simulink model "npc_controller"  (R2022a)
settings: Solver=FixedStepDiscrete  StartTime=0.0  StopTime=20  RelTol=1e-3  EnableMultiTasking=on
undefined symbols (not defined in the file): CAN_O_INT, CANA_BASE, Down, GPTRIP1SEL, GPTRIP2SEL, GPTRIP3SEL, Tsw, TZ1, TZ2, TZ3, Up
libraries: simulink x147, hdlsllib x90, c2802xlib x34, c2837xDlib x20, c280xlib x12, canmsglib x9, c2838xlib x8, idelinklib_common x3, c2806xlib x2, slpidlib x2, c28004xlib x2, c281xlib x2
(part 10 of 42)

== system npc_controller/CONTROL/STATE-MACHINE/CPU_CONTROL_750_precharge_pfc_ok2/updateSequencePhA ==
  note: Notes:
      | vac_adc = vac_actual*0.00264706+1.65
      | iac_adc = iac_actual*0.02+1.65
      | vbulk_adc = vbulk_actual*3.49e-3
      | vmid_adc = vmid_acutal*3.49e-3
  note: Note:
      | Vmid         C2
      | Vbulk        A5
      |
      | Va            A2/B6
      | Vb            B0
      | Vc            C0
      |
      | Ia             A3
      | Ib             A10/B1, C10
      | Ic             C1
  vxn : Inport
  ix : Inport  Port=2
  f : TriggerPort  TriggerType=function-call  VariantControl=(inherit)
      settings: CopyFcn=Stateflow.SLINSF.SimulinkMan.removeBlockPreDeleteFcn  PreDeleteFcn=Stateflow.SLINSF.SimulinkMan.unsafePredeleteFcn
  Cast To Single : DataTypeConversion  Commented=on  OutDataTypeStr=single  SaturateOnIntegerOverflow=off  RndMeth=Floor
  Cast To Single1 : DataTypeConversion  Commented=on  OutDataTypeStr=single  SaturateOnIntegerOverflow=off  RndMeth=Floor
  From5 : From  Commented=on  GotoTag=vxn
  From6 : From  Commented=on  GotoTag=pol_vxn
  From7 : From  Commented=on  GotoTag=ix
  From8 : From  Commented=on  GotoTag=pol_ix
  Function-Call Generator : simulink/Ports & Subsystems/Function-Call Generator  sample_time=-1  numberOfIterations=1  DisallowWideOutput=off
  Function-Call Split : FunctionCallSplit  NumOutputPorts=2
  Function-Call Split2 : FunctionCallSplit  NumOutputPorts=2
  Gain2 : Gain  Commented=on  Gain=200
  Gain3 : Gain  Commented=on  Gain=200
  Mux : Mux  Commented=on  Inputs=2
  Mux1 : Mux  Commented=on  Inputs=2
  Scope : Scope  Commented=on  NumInputPorts=3
  pol_final1 : Subsystem  Commented=on
  pol_ix1 : Subsystem  Commented=on
  pol_vxn1 : Subsystem
  vx_seq : Outport
  wires:
  pol_vxn1/1(pol_vxn) -> [pol_vxn]
  [pol_vxn] -> vx_seq/1
  Gain3/1 -> Mux1/2
  Cast To Single1/1 -> Gain3/1
  Gain2/1 -> Mux/2
  From7/1 -> Mux1/1
  From5/1 -> Mux/1
  ix/1 -> [ix]
  Cast To Single/1 -> Gain2/1
  From8/1 -> Cast To Single1/1
  From6/1 -> Cast To Single/1
  Mux1/1 -> Scope/2
  Mux/1 -> Scope/1
  pol_final1/1(pol) -> Scope/3
  [pol_ix] -> pol_final1/2(ix)
  [pol_vxn] -> pol_final1/1(vxn)
  pol_ix1/1(pol_ix) -> [pol_ix]
  [ix] -> pol_ix1/1(ix)
  [vxn] -> pol_vxn1/1(vxn)
  Function-Call Split2/2 -> Function-Call Split/1
  Function-Call Generator/1 -> Function-Call Split2/1
  Function-Call Split/1 -> pol_ix1/Trigger
  Function-Call Split2/1 -> pol_vxn1/Trigger
  Function-Call Split/2 -> pol_final1/Trigger
  vxn/1 -> [vxn]

== system npc_controller/CONTROL/STATE-MACHINE/CPU_CONTROL_750_precharge_pfc_ok2/updateSequencePhB ==
  note: Note:
      |
      | Function PWM # GPIO # LAUNCHPAD PIN #
      |
      | Synci EPWM1A GPIO0 J4.40
      | EPWM1B GPIO1 J4.39
      |
      | ORPS EPMW2A GPIO2 J4.38
      | EPWM2B GPIO3 J4.37
      |
      | RELAY EPWM3A GPIO4 J4.36
      |
      | TZ GPIO62 XX
      |
      | a_s1 EPWM6A GPIO10 J8.76
      | a_s2 EPWM7B GPIO13 XX
      | a_s3 EPWM6B GPIO11 J8.75
      | a_s4 EPWM7A GPIO12 XX
      |
      | b_s1 EPWM8B GPIO15 J8.73
      | b_s2 EPWM9B GPIO17 XX
      | b_s3 EPWM8A GPIO14 J8.74
      | b_s4 EPWM9A GPIO16 J4.33
      |
      | c_s1 EPWM10B GPIO19 J1.3
      | c_s2 EPWM11B GPIO21 XX
      | c_s3 EPWM10A GPIO18 J1.4
      | c_s4 EPWM11A GPIO20 XX
  note: Notes:
      | vac_adc = vac_actual*0.00264706+1.65
      | iac_adc = iac_actual*0.02+1.65
      | vbulk_adc = vbulk_actual*3.49e-3
      | vmid_adc = vmid_acutal*3.49e-3
  note: Note:
      | Vmid         C2
      | Vbulk        A5
      |
      | Va            A2/B6
      | Vb            B0
      | Vc            C0
      |
      | Ia             A3
      | Ib             A10/B1, C10
      | Ic             C1
  vxn : Inport
  ix : Inport  Port=2
  f : TriggerPort  TriggerType=function-call  VariantControl=(inherit)
      settings: CopyFcn=Stateflow.SLINSF.SimulinkMan.removeBlockPreDeleteFcn  PreDeleteFcn=Stateflow.SLINSF.SimulinkMan.unsafePredeleteFcn
  Cast To Single : DataTypeConversion  Commented=on  OutDataTypeStr=single  SaturateOnIntegerOverflow=off  RndMeth=Floor
  Cast To Single1 : DataTypeConversion  Commented=on  OutDataTypeStr=single  SaturateOnIntegerOverflow=off  RndMeth=Floor
  From5 : From  Commented=on  GotoTag=vxn
  From6 : From  Commented=on  GotoTag=pol_vxn
  From7 : From  Commented=on  GotoTag=ix
  From8 : From  Commented=on  GotoTag=pol_ix
  Function-Call Generator : simulink/Ports & Subsystems/Function-Call Generator  sample_time=-1  numberOfIterations=1  DisallowWideOutput=off
  Function-Call Split : FunctionCallSplit  NumOutputPorts=2
  Function-Call Split2 : FunctionCallSplit  NumOutputPorts=2
  Gain2 : Gain  Commented=on  Gain=200
  Gain3 : Gain  Commented=on  Gain=200
  Mux : Mux  Commented=on  Inputs=2
  Mux1 : Mux  Commented=on  Inputs=2
  Scope : Scope  Commented=on  NumInputPorts=3
  pol_final1 : Subsystem  Commented=on
  pol_ix1 : Subsystem  Commented=on
  pol_vxn1 : Subsystem
  vx_seq : Outport
  wires:
  pol_vxn1/1(pol_vxn) -> [pol_vxn]
  [pol_vxn] -> vx_seq/1
  Gain3/1 -> Mux1/2
  Cast To Single1/1 -> Gain3/1
  Gain2/1 -> Mux/2
  From7/1 -> Mux1/1
  From5/1 -> Mux/1
  ix/1 -> [ix]
  Cast To Single/1 -> Gain2/1
  From8/1 -> Cast To Single1/1
  From6/1 -> Cast To Single/1
  Mux1/1 -> Scope/2
  Mux/1 -> Scope/1
  pol_final1/1(pol) -> Scope/3
  [pol_ix] -> pol_final1/2(ix)
  [pol_vxn] -> pol_final1/1(vxn)
  pol_ix1/1(pol_ix) -> [pol_ix]
  [ix] -> pol_ix1/1(ix)
  [vxn] -> pol_vxn1/1(vxn)
  Function-Call Split2/2 -> Function-Call Split/1
  Function-Call Generator/1 -> Function-Call Split2/1
  Function-Call Split/1 -> pol_ix1/Trigger
  Function-Call Split2/1 -> pol_vxn1/Trigger
  Function-Call Split/2 -> pol_final1/Trigger
  vxn/1 -> [vxn]

== system npc_controller/CONTROL/STATE-MACHINE/CPU_CONTROL_750_precharge_pfc_ok2/updateSequencePhC ==
  note: Note:
      |
      | Function PWM # GPIO # LAUNCHPAD PIN #
      |
      | Synci EPWM1A GPIO0 J4.40
      | EPWM1B GPIO1 J4.39
      |
      | ORPS EPMW2A GPIO2 J4.38
      | EPWM2B GPIO3 J4.37
      |
      | RELAY EPWM3A GPIO4 J4.36
      |
      | TZ GPIO62 XX
      |
      | a_s1 EPWM6A GPIO10 J8.76
      | a_s2 EPWM7B GPIO13 XX
      | a_s3 EPWM6B GPIO11 J8.75
      | a_s4 EPWM7A GPIO12 XX
      |
      | b_s1 EPWM8B GPIO15 J8.73
      | b_s2 EPWM9B GPIO17 XX
      | b_s3 EPWM8A GPIO14 J8.74
      | b_s4 EPWM9A GPIO16 J4.33
      |
      | c_s1 EPWM10B GPIO19 J1.3
      | c_s2 EPWM11B GPIO21 XX
      | c_s3 EPWM10A GPIO18 J1.4
      | c_s4 EPWM11A GPIO20 XX
  note: Notes:
      | vac_adc = vac_actual*0.00264706+1.65
      | iac_adc = iac_actual*0.02+1.65
      | vbulk_adc = vbulk_actual*3.49e-3
      | vmid_adc = vmid_acutal*3.49e-3
  note: Note:
      | Vmid         C2
      | Vbulk        A5
      |
      | Va            A2/B6
      | Vb            B0
      | Vc            C0
      |
      | Ia             A3
      | Ib             A10/B1, C10
      | Ic             C1
  vxn : Inport
  ix : Inport  Port=2
  f : TriggerPort  TriggerType=function-call  VariantControl=(inherit)
      settings: CopyFcn=Stateflow.SLINSF.SimulinkMan.removeBlockPreDeleteFcn  PreDeleteFcn=Stateflow.SLINSF.SimulinkMan.unsafePredeleteFcn
  Cast To Single : DataTypeConversion  Commented=on  OutDataTypeStr=single  SaturateOnIntegerOverflow=off  RndMeth=Floor
  Cast To Single1 : DataTypeConversion  Commented=on  OutDataTypeStr=single  SaturateOnIntegerOverflow=off  RndMeth=Floor
  From5 : From  Commented=on  GotoTag=vxn
  From6 : From  Commented=on  GotoTag=pol_vxn
  From7 : From  Commented=on  GotoTag=ix
  From8 : From  Commented=on  GotoTag=pol_ix
  Function-Call Generator : simulink/Ports & Subsystems/Function-Call Generator  sample_time=-1  numberOfIterations=1  DisallowWideOutput=off
  Function-Call Split : FunctionCallSplit  NumOutputPorts=2
  Function-Call Split2 : FunctionCallSplit  NumOutputPorts=2
  Gain2 : Gain  Commented=on  Gain=200
  Gain3 : Gain  Commented=on  Gain=200
  Mux : Mux  Commented=on  Inputs=2
  Mux1 : Mux  Commented=on  Inputs=2
  Scope : Scope  Commented=on  NumInputPorts=3
  pol_final1 : Subsystem  Commented=on
  pol_ix1 : Subsystem  Commented=on
  pol_vxn1 : Subsystem
  vx_seq : Outport
  wires:
  [pol_vxn] -> vx_seq/1
  Gain3/1 -> Mux1/2
  Cast To Single1/1 -> Gain3/1
  Gain2/1 -> Mux/2
  From7/1 -> Mux1/1
  From5/1 -> Mux/1
  ix/1 -> [ix]
  Cast To Single/1 -> Gain2/1
  From8/1 -> Cast To Single1/1
  From6/1 -> Cast To Single/1
  Mux1/1 -> Scope/2
  Mux/1 -> Scope/1
  pol_final1/1(pol) -> Scope/3
  [pol_ix] -> pol_final1/2(ix)
  [pol_vxn] -> pol_final1/1(vxn)
  pol_ix1/1(pol_ix) -> [pol_ix]
  [ix] -> pol_ix1/1(ix)
  pol_vxn1/1(pol_vxn) -> [pol_vxn]
  [vxn] -> pol_vxn1/1(vxn)
  Function-Call Split2/2 -> Function-Call Split/1
  Function-Call Generator/1 -> Function-Call Split2/1
  Function-Call Split/1 -> pol_ix1/Trigger
  Function-Call Split2/1 -> pol_vxn1/Trigger
  Function-Call Split/2 -> pol_final1/Trigger
  vxn/1 -> [vxn]

== system npc_controller/CONTROL/STATE-MACHINE/If Action Subsystem ==
  Action Port : ActionPort
  Constant3 : Constant  Value=0  OutDataTypeStr=single  SampleTime=-1
  Out1 : Outport
  wires:
  Constant3/1 -> Out1/1

== system npc_controller/CONTROL/STATE-MACHINE/If Action Subsystem1 ==
  Action Port : ActionPort
  Constant3 : Constant  Value=2048  OutDataTypeStr=single  SampleTime=-1
  Out1 : Outport
  wires:
  Constant3/1 -> Out1/1

== system npc_controller/CONTROL/STATE-MACHINE/PLL ==
  note: Voltage-Controlled Oscillator (VCO)
  note: Loop Filter (LF)
  note: Phase Detector (PD)
  vxn : Inport  OutDataTypeStr=single
  Data Store Write : DataStoreWrite  Commented=on  DataStoreName=theta  IndexOptions=Index vector (dialog)  Indices=1  OutputSizes=1
  Delay1 : Delay  DelayLength=1  StateName=mem2
  Delay2 : Delay  DelayLength=1  StateName=mem1
  Gain : Gain  Commented=on  Gain=100  ParamDataTypeStr=uint16  OutDataTypeStr=uint16
  Gain4 : Gain  Gain=1/(2*pi)  ParamDataTypeStr=single  OutDataTypeStr=single
  Integrator2 : Subsystem
  Product : Product  OutDataTypeStr=single
  Product1 : Product  OutDataTypeStr=single
  Product2 : Product  OutDataTypeStr=single
  Scope1 : Scope  NumInputPorts=3
  Scope2 : Scope  NumInputPorts=4
  Scope4 : Scope  NumInputPorts=3
  Scope5 : Scope  NumInputPorts=3
  Subsystem1 : Subsystem
  Subsystem2 : Subsystem
  Sum : Sum  Inputs=|+-  AccumDataTypeStr=single  OutDataTypeStr=single
  Trigonometric Function1 : Trigonometry  Operator=sincos
  freq1 : Outport  VectorParamsAs1DForOutWhenUnconnected=off
  angle : Outport  Port=2  VectorParamsAs1DForOutWhenUnconnected=off
  mag1 : Outport  Port=3  VectorParamsAs1DForOutWhenUnconnected=off
  wires:
  Integrator2/1(theta) -> Scope2/3, angle/1, Gain/1, Delay1/1
  Subsystem1/1(y) -> mag1/1, Scope2/4, Product1/1, Scope4/1
  Sum/1 -> Scope1/3, Product2/1, Scope5/1, Delay2/1
  Gain4/1 -> freq1/1, Scope2/2
  Gain/1 -> Data Store Write/1
  vxn/1 -> Scope2/1, Scope1/1, Sum/1
  Product/1 -> Subsystem1/1(u)
  Product1/1 -> Scope4/3, Scope1/2, Sum/2
  Trigonometric Function1/2 -> Scope5/2, Product2/2
  Delay2/1 -> Product/1
  Subsystem2/1(y) -> Gain4/1, Integrator2/1(omega)
  Product2/1 -> Subsystem2/1(u), Scope5/3
  Delay1/1 -> Trigonometric Function1/1
  Trigonometric Function1/1 -> Scope4/2, Product1/2, Product/2

== system npc_controller/CONTROL/STATE-MACHINE/Subsystem1 ==
  adc : Inport
  Less Than : RelationalOperator  Operator=>  OutDataTypeStr=boolean  RndMeth=Simplest  InputSameDT=off
  Less Than1 : RelationalOperator  Operator=<  OutDataTypeStr=boolean  RndMeth=Simplest  InputSameDT=off
  Offset7 : Constant  Value=0  OutDataTypeStr=single
  Offset8 : Constant  Value=0  OutDataTypeStr=single
  Product : Product  OutDataTypeStr=single
  Product1 : Product  OutDataTypeStr=single
  vabc7 : Sum  Inputs=|+-  AccumDataTypeStr=single  OutDataTypeStr=single
  adc_rect : Outport
  wires:
  vabc7/1 -> adc_rect/1
  adc/1 -> Less Than/1, Product/1, Less Than1/1, Product1/1
  Product1/1 -> vabc7/2
  Product/1 -> vabc7/1
  Less Than/1 -> Product/2
  Offset8/1 -> Less Than1/2
  Offset7/1 -> Less Than/2
  Less Than1/1 -> Product1/2

== system npc_controller/CONTROL/STATE-MACHINE/Update_PFC_EN ==
  Dig_Input : Inport  OutDataTypeStr=boolean
  Constant : Constant  Value=67  OutDataTypeStr=uint16
  Constant1 : Constant  Value=67  OutDataTypeStr=uint16
  Constant2 : Constant  OutDataTypeStr=boolean
  Validate_DI : MATLABSystem  System=Validate_DI  SimulateUsing=Code generation
      mask Type: Validate_DI
      mask Display:
      | disp('Validate_DI');
      | port_label('input',1,'din');
      | port_label('input',2,'assert_logic');
      | port_label('input',3,'assert_dly');
      | port_label('input',4,'deassert_dly');
      | port_label('output',1,'status');
  Dig_Input_State : Outport  OutDataTypeStr=boolean
  wires:
  Constant1/1 -> Validate_DI/4
  Constant/1 -> Validate_DI/3
  Dig_Input/1 -> Validate_DI/1
  Constant2/1 -> Validate_DI/2
  Validate_DI/1 -> Dig_Input_State/1

== system npc_controller/CONTROL/SVPWM/IIR Filter1 ==
  x[n] : Inport
  1 - Lambda : Gain  Gain=1 - 0.98
  Delay : Delay  DelayLength=1
  Lambda : Gain  Gain=0.98
  Sum : Sum  Inputs=|++
  y[n] : Outport
  wires:
  x[n]/1 -> 1 - Lambda/1
  1 - Lambda/1 -> Sum/1
  Sum/1 -> Delay/1, y[n]/1
  Lambda/1 -> Sum/2
  Delay/1 -> Lambda/1

== system npc_controller/CONTROL/SVPWM/IIR Filter2 ==
  x[n] : Inport
  1 - Lambda : Gain  Gain=1 - 0.98
  Delay : Delay  DelayLength=1
  Lambda : Gain  Gain=0.98
  Sum : Sum  Inputs=|++
  y[n] : Outport
  wires:
  Delay/1 -> Lambda/1
  Lambda/1 -> Sum/2
  Sum/1 -> y[n]/1, Delay/1
  1 - Lambda/1 -> Sum/1
  x[n]/1 -> 1 - Lambda/1

== system npc_controller/CONTROL/SVPWM/PLL_Block ==
  abc : Inport
  Demux : Demux  Commented=on  Outputs=3
  If1 : If  Commented=on  IfExpression=(u1 > 0)  ShowElse=off
  SRF_PLL : Subsystem
  Subsystem : Subsystem  Commented=on
  theta : Outport  OutDataTypeStr=single
  wires:
  Demux/1 -> Subsystem/1(In1)
  abc/1 -> Demux/1, SRF_PLL/1(Vabc)
  Subsystem/1(Out1) -> If1/1
  SRF_PLL/3(theta) -> theta/1

== system npc_controller/CONTROL/SVPWM/SVPWM Generator (3-Level)1 ==
  Vabc_ref : Inport
  Vdc_P0 : Inport  Port=2
  Vdc_0N : Inport  Port=3
  Idc : Inport  Port=4
  Kp : Inport  Port=5
  Fsw : Inport  Port=6
  Neutral Point Voltage Deviation Control System : Subsystem
  Selector2 : Selector  InputPortWidth=2  IndexOptions=Index vector (dialog)  Indices=1  OutputSizes=1
  Timing Calculation : Subsystem
  TgABC_On : Outport
  TgABC_Off : Outport  Port=2
  Sn : Outport  Port=3
  wires:
  Fsw/1 -> Timing Calculation/3(Fsw)
  Kp/1 -> Neutral Point Voltage Deviation Control System/4(Kp)
  Vdc_0N/1 -> Neutral Point Voltage Deviation Control System/2(Vdc_0N)
  Vabc_ref/1 -> Timing Calculation/1(Uref)
  Neutral Point Voltage Deviation Control System/1(Out) -> Timing Calculation/2(DeltaVdc)
  Timing Calculation/3(Sn) -> Selector2/1
  Selector2/1 -> Sn/1
  Timing Calculation/1(TgABC_On) -> TgABC_On/1
  Timing Calculation/2(TgABC_Off) -> TgABC_Off/1
  Idc/1 -> Neutral Point Voltage Deviation Control System/3(Idc)
  Vdc_P0/1 -> Neutral Point Voltage Deviation Control System/1(Vdc_P0)

== system npc_controller/CONTROL/SVPWM/SVPWM2/calcCmpBal ==
  r_seq : Inport  OutDataTypeStr=double  PortDimensions=4
  s_seq : Inport  Port=2  OutDataTypeStr=double  PortDimensions=4
  t_seq : Inport  Port=3  OutDataTypeStr=double  PortDimensions=4
  Tx : Inport  Port=4  OutDataTypeStr=double  PortDimensions=1
  Ty : Inport  Port=5  OutDataTypeStr=double  PortDimensions=1
  Tz : Inport  Port=6  OutDataTypeStr=double  PortDimensions=1
  vbal_coef : Inport  Port=7
  f : TriggerPort  TriggerType=function-call  VariantControl=(inherit)
      settings: CopyFcn=Stateflow.SLINSF.SimulinkMan.removeBlockPreDeleteFcn  PreDeleteFcn=Stateflow.SLINSF.SimulinkMan.unsafePredeleteFcn
  Add : Sum  Inputs=++++
  Add1 : Sum  Inputs=++++
  Add2 : Sum  Inputs=++++
  Constant : Constant
  Demux : Demux
  Demux1 : Demux
  Demux2 : Demux
  Display : Display
  Display1 : Display
  Gain1 : Gain  Gain=1/15e-6
  Gain11 : Gain  Gain=1/15e-6
  Gain6 : Gain  Gain=1/15e-6
  Product{,1..17} (18 alike) : Product
  Subtract : Sum  Inputs=+-
  cmp_r : Outport
  cmp_s : Outport  Port=2
  cmp_t : Outport  Port=3
  wires:
  [vbal_coef_n] -> Product14/2
  [vbal_coef_p] -> Product15/2
  [vbal_coef_p] -> Product17/2
  [vbal_coef_n] -> Product16/2
  [vbal_coef_n] -> Product13/2
  [vbal_coef_p] -> Product12/2
  vbal_coef/1 -> [vbal_coef_p], Display1/1, Subtract/2
  Subtract/1 -> [vbal_coef_n], Display/1
  Constant/1 -> Subtract/1
  Tz/1 -> [Tz]
  s_seq/1 -> [s_seq]
  t_seq/1 -> [t_seq]
  Gain11/1 -> cmp_t/1
  Product17/1 -> Product11/2
  [Ty] -> Product10/2
  [Tx] -> Product9/2
  Demux2/4 -> Product11/1
  Demux2/3 -> Product10/1
  Demux2/2 -> Product9/1
  Product11/1 -> Add2/4
  Product10/1 -> Add2/3
  Product9/1 -> Add2/2
  Demux2/1 -> Product8/1
  Product16/1 -> Product8/2
  Product8/1 -> Add2/1
  [Tz] -> Product17/1
  Add2/1 -> Gain11/1
  [Tz] -> Product16/1
  [t_seq] -> Demux2/1
  Gain6/1 -> cmp_s/1
  [s_seq] -> Demux1/1
  [Tz] -> Product14/1
  Add1/1 -> Gain6/1
  [Tz] -> Product15/1
  Product4/1 -> Add1/1
  Product14/1 -> Product4/2
  Demux1/1 -> Product4/1
  Product5/1 -> Add1/2
  Product6/1 -> Add1/3
  Product7/1 -> Add1/4
  Demux1/2 -> Product5/1
  Demux1/3 -> Product6/1
  Demux1/4 -> Product7/1
  [Tx] -> Product5/2
  [Ty] -> Product6/2
  Product15/1 -> Product7/2
  Product12/1 -> Product3/2
  [Ty] -> Product2/2
  [Tx] -> Product1/2
  Demux/4 -> Product3/1
  Demux/3 -> Product2/1
  Demux/2 -> Product1/1
  Product3/1 -> Add/4
  Product2/1 -> Add/3
  Product1/1 -> Add/2
  Demux/1 -> Product/1
  Product13/1 -> Product/2
  Product/1 -> Add/1
  [Tz] -> Product12/1
  Gain1/1 -> cmp_r/1
  Add/1 -> Gain1/1
  [Tz] -> Product13/1
  [r_seq] -> Demux/1
  Tx/1 -> [Tx]
  Ty/1 -> [Ty]
  r_seq/1 -> [r_seq]

== system npc_controller/CONTROL/SVPWM/SVPWM2/calcDwellingTimes ==
  Tsw : Inport  OutDataTypeStr=double  PortDimensions=1
  vref_fict_mag_alpha : Inport  Port=2  OutDataTypeStr=double  PortDimensions=1
  vref_fict_mag_beta : Inport  Port=3  OutDataTypeStr=double  PortDimensions=1
  vx_fict_mag_alpha : Inport  Port=4  OutDataTypeStr=double  PortDimensions=1
  vx_fict_mag_beta : Inport  Port=5  OutDataTypeStr=double  PortDimensions=1
  vy_fict_mag_alpha : Inport  Port=6  OutDataTypeStr=double  PortDimensions=1
  vy_fict_mag_beta : Inport  Port=7  OutDataTypeStr=double  PortDimensions=1
  f : TriggerPort  TriggerType=function-call  VariantControl=(inherit)
      settings: CopyFcn=Stateflow.SLINSF.SimulinkMan.removeBlockPreDeleteFcn  PreDeleteFcn=Stateflow.SLINSF.SimulinkMan.unsafePredeleteFcn
  Add : Sum  Inputs=+-
  Add1 : Sum  Inputs=+--
  Cast To Single : DataTypeConversion  OutDataTypeStr=single  SaturateOnIntegerOverflow=off  RndMeth=Floor
  Cast To Single1 : DataTypeConversion  OutDataTypeStr=single  SaturateOnIntegerOverflow=off  RndMeth=Floor
  Cast To Single2 : DataTypeConversion  OutDataTypeStr=single  SaturateOnIntegerOverflow=off  RndMeth=Floor
  Display{,1..17} (18 alike) : Display
  Divide : Product  Inputs=**/
  Divide1 : Product  Inputs=*/
  Product{,1..5} (6 alike) : Product
  Subtract : Sum  Inputs=+-
  Subtract1 : Sum  Inputs=+-
  Tx : Outport
  Ty : Outport  Port=2
  Tz : Outport  Port=3
  wires:
  Add1/1 -> Display3/1, Cast To Single2/1
  Divide1/1 -> Display2/1, [Ty], Cast To Single1/1
  Divide/1 -> Cast To Single/1, Display1/1, [Tx]
  Tsw/1 -> Display4/1, [Tsw]
  vref_fict_mag_alpha/1 -> Display5/1, [vref_fict_mag_alpha]
  vref_fict_mag_beta/1 -> Display6/1, [vref_fict_mag_beta]
  vx_fict_mag_alpha/1 -> Display7/1, [vx_fict_mag_alpha]
  vx_fict_mag_beta/1 -> Display8/1, [vx_fict_mag_beta]
  vy_fict_mag_alpha/1 -> Display9/1, [vy_fict_mag_alpha]
  vy_fict_mag_beta/1 -> Display10/1, [vy_fict_mag_beta]
  [vref_fict_mag_beta] -> Product/1
  [vy_fict_mag_alpha] -> Product/2
  [vref_fict_mag_alpha] -> Product1/1
  [vy_fict_mag_beta] -> Product1/2
  [vx_fict_mag_alpha] -> Product3/1
  [vy_fict_mag_beta] -> Product3/2
  Product/1 -> Add/1, Display12/1
  Product1/1 -> Add/2, Display13/1
  Product2/1 -> Subtract/1, Display15/1
  Product3/1 -> Subtract/2, Display14/1
  Add/1 -> Divide/2, Display11/1
  Subtract/1 -> Divide/3, Display16/1
  Product4/1 -> Display/1, Subtract1/1
  [vref_fict_mag_alpha] -> Product4/1
  [Tsw] -> Product4/2
  [vx_fict_mag_alpha] -> Product5/1
  [Tx] -> Product5/2
  Product5/1 -> Subtract1/2
  Subtract1/1 -> Divide1/1
  [vy_fict_mag_alpha] -> Divide1/2
  [Ty] -> Add1/3
  [Tx] -> Add1/2
  [Tsw] -> Add1/1
  Cast To Single/1 -> Tx/1
  Cast To Single1/1 -> Ty/1
  Cast To Single2/1 -> Tz/1
  [Tsw] -> Divide/1, Display17/1
  [vy_fict_mag_alpha] -> Product2/2
  [vx_fict_mag_beta] -> Product2/1

== system npc_controller/CONTROL/SVPWM/SVPWM2/detSeq ==
  subsector : Inport  OutDataTypeStr=double  PortDimensions=1
  f : TriggerPort  TriggerType=function-call  VariantControl=(inherit)
      settings: CopyFcn=Stateflow.SLINSF.SimulinkMan.removeBlockPreDeleteFcn  PreDeleteFcn=Stateflow.SLINSF.SimulinkMan.unsafePredeleteFcn
  Cast To Double : DataTypeConversion  OutDataTypeStr=double  SaturateOnIntegerOverflow=off  RndMeth=Floor
  Cast To Double1 : DataTypeConversion  OutDataTypeStr=double  SaturateOnIntegerOverflow=off  RndMeth=Floor
  Cast To Double2 : DataTypeConversion  OutDataTypeStr=double  SaturateOnIntegerOverflow=off  RndMeth=Floor
  Constant{,5,7..8,12,17} (6 alike) : Constant  Value=[0 1 1 1]
  Constant1 : Constant  Value=[0 1 0 1]
  Constant{2..3,10..11,14..15} (6 alike) : Constant  Value=[0 0 0 1]
  Constant13 : Constant  Value=[0 1 0 1]
  Constant16 : Constant  Value=[0 0 1 1]
  Constant18 : Constant  Commented=on  Value=[1 1 0 0]
  Constant19 : Constant  Commented=on  Value=[1 0 0 0]
  Constant20 : Constant  Commented=on  Value=[1 1 1 0]
  Constant21 : Constant  Commented=on  Value=[1 1 1 0]
  Constant22 : Constant  Commented=on  Value=[1 1 0 0]
  Constant23 : Constant  Commented=on  Value=[1 0 0 0]
  Constant24 : Constant  Commented=on  Value=[1 0 0 0]
  Constant25 : Constant  Commented=on  Value=[1 1 1 0]
  Constant26 : Constant  Commented=on  Value=[1 1 0 0]
  Constant4 : Constant  Value=[0 0 1 1]
  Constant6 : Constant  Value=[0 0 1 1]
  Constant9 : Constant  Value=[0 1 0 1]
  Multiport Switch : MultiPortSwitch  Inputs=6  DataPortForDefault=Additional data port  SaturateOnIntegerOverflow=off  InputSameDT=off
  Multiport Switch1 : MultiPortSwitch  Inputs=6  DataPortForDefault=Additional data port  SaturateOnIntegerOverflow=off  InputSameDT=off
  Multiport Switch2 : MultiPortSwitch  Inputs=6  DataPortForDefault=Additional data port  SaturateOnIntegerOverflow=off  InputSameDT=off
  r_seq : Outport
  s_seq : Outport  Port=2
  t_seq : Outport  Port=3
  wires:
  Multiport Switch2/1 -> Cast To Double2/1
  Constant15/1 -> Multiport Switch2/3
  Constant16/1 -> Multiport Switch2/4
  Constant17/1 -> Multiport Switch2/5
  Constant12/1 -> Multiport Switch2/6
  Constant13/1 -> Multiport Switch2/7
  Constant14/1 -> Multiport Switch2/2
  [subsector] -> Multiport Switch2/1
  Multiport Switch1/1 -> Cast To Double1/1
  [subsector] -> Multiport Switch1/1
  Constant6/1 -> Multiport Switch1/2
  Constant11/1 -> Multiport Switch1/7
  Constant10/1 -> Multiport Switch1/6
  Constant9/1 -> Multiport Switch1/5
  Constant8/1 -> Multiport Switch1/4
  Constant7/1 -> Multiport Switch1/3
  Constant1/1 -> Multiport Switch/3
  Constant2/1 -> Multiport Switch/4
  Constant3/1 -> Multiport Switch/5
  Constant4/1 -> Multiport Switch/6
  Constant5/1 -> Multiport Switch/7
  Constant/1 -> Multiport Switch/2
  [subsector] -> Multiport Switch/1
  subsector/1 -> [subsector]
  Multiport Switch/1 -> Cast To Double/1
  Cast To Double/1 -> r_seq/1
  Cast To Double1/1 -> s_seq/1
  Cast To Double2/1 -> t_seq/1

== system npc_controller/CONTROL/SVPWM/SVPWM_with_bal/calcCmp ==
  r_seq : Inport  OutDataTypeStr=double  PortDimensions=4
  s_seq : Inport  Port=2  OutDataTypeStr=double  PortDimensions=4
  t_seq : Inport  Port=3  OutDataTypeStr=double  PortDimensions=4
  Tx : Inport  Port=4  OutDataTypeStr=double  PortDimensions=1
  Ty : Inport  Port=5  OutDataTypeStr=double  PortDimensions=1
  Tz : Inport  Port=6  OutDataTypeStr=double  PortDimensions=1
  f : TriggerPort  TriggerType=function-call  VariantControl=(inherit)
      settings: CopyFcn=Stateflow.SLINSF.SimulinkMan.removeBlockPreDeleteFcn  PreDeleteFcn=Stateflow.SLINSF.SimulinkMan.unsafePredeleteFcn
  Add : Sum  Inputs=++++
  Add1 : Sum  Inputs=++++
  Add2 : Sum  Inputs=++++
  Demux : Demux
  Demux1 : Demux
  Demux2 : Demux
  Gain{,2,5,7,10,12} (6 alike) : Gain  Gain=0.5
  Gain1 : Gain  Gain=1/15e-6
  Gain11 : Gain  Gain=1/15e-6
  Gain6 : Gain  Gain=1/15e-6
  Product{,1..11} (12 alike) : Product
  cmp_r : Outport
  cmp_s : Outport  Port=2
  cmp_t : Outport  Port=3
  wires:
  r_seq/1 -> [r_seq]
  Ty/1 -> [Ty]
  Tx/1 -> [Tx]
  Tz/1 -> [Tz]
  [r_seq] -> Demux/1
  [Tz] -> Gain/1
  Add/1 -> Gain1/1
  Gain1/1 -> cmp_r/1
  [Tz] -> Gain2/1
  Product/1 -> Add/1
  Gain/1 -> Product/2
  Demux/1 -> Product/1
  Product1/1 -> Add/2
  Product2/1 -> Add/3
  Product3/1 -> Add/4
  Demux/2 -> Product1/1
  Demux/3 -> Product2/1
  Demux/4 -> Product3/1
  [Tx] -> Product1/2
  [Ty] -> Product2/2
  Gain2/1 -> Product3/2
  Gain7/1 -> Product7/2
  [Ty] -> Product6/2
  [Tx] -> Product5/2
  Demux1/4 -> Product7/1
  Demux1/3 -> Product6/1
  Demux1/2 -> Product5/1
  Product7/1 -> Add1/4
  Product6/1 -> Add1/3
  Product5/1 -> Add1/2
  Demux1/1 -> Product4/1
  Gain5/1 -> Product4/2
  Product4/1 -> Add1/1
  [Tz] -> Gain7/1
  Add1/1 -> Gain6/1
  [Tz] -> Gain5/1
  [s_seq] -> Demux1/1
  Gain6/1 -> cmp_s/1
  [t_seq] -> Demux2/1
  [Tz] -> Gain10/1
  Add2/1 -> Gain11/1
  [Tz] -> Gain12/1
  Product8/1 -> Add2/1
  Gain10/1 -> Product8/2
  Demux2/1 -> Product8/1
  Product9/1 -> Add2/2
  Product10/1 -> Add2/3
  Product11/1 -> Add2/4
  Demux2/2 -> Product9/1
  Demux2/3 -> Product10/1
  Demux2/4 -> Product11/1
  [Tx] -> Product9/2
  [Ty] -> Product10/2
  Gain12/1 -> Product11/2
  Gain11/1 -> cmp_t/1
  t_seq/1 -> [t_seq]
  s_seq/1 -> [s_seq]

== system npc_controller/CONTROL/SVPWM/SVPWM_with_bal/calcCmpWithBal ==
  r_seq : Inport  OutDataTypeStr=double  PortDimensions=4
  s_seq : Inport  Port=2  OutDataTypeStr=double  PortDimensions=4
  t_seq : Inport  Port=3  OutDataTypeStr=double  PortDimensions=4
  Tx : Inport  Port=4  OutDataTypeStr=double  PortDimensions=1
  Ty : Inport  Port=5  OutDataTypeStr=double  PortDimensions=1
  Tz : Inport  Port=6  OutDataTypeStr=double  PortDimensions=1
  f : TriggerPort  TriggerType=function-call  VariantControl=(inherit)
      settings: CopyFcn=Stateflow.SLINSF.SimulinkMan.removeBlockPreDeleteFcn  PreDeleteFcn=Stateflow.SLINSF.SimulinkMan.unsafePredeleteFcn
  Add : Sum  Inputs=++++
  Add1 : Sum  Inputs=++++
  Add2 : Sum  Inputs=++++
  Demux : Demux
  Demux1 : Demux
  Demux2 : Demux
  Gain{,2,5,7,10,12} (6 alike) : Gain  Gain=0.5
  Gain1 : Gain  Gain=1/15e-6
  Gain11 : Gain  Gain=1/15e-6
  Gain6 : Gain  Gain=1/15e-6
  Product{,1..11} (12 alike) : Product
  cmp_r : Outport
  cmp_s : Outport  Port=2
  cmp_t : Outport  Port=3
  wires:
  r_seq/1 -> [r_seq]
  Ty/1 -> [Ty]
  Tx/1 -> [Tx]
  Tz/1 -> [Tz]
  [r_seq] -> Demux/1
  [Tz] -> Gain/1
  Add/1 -> Gain1/1
  Gain1/1 -> cmp_r/1
  [Tz] -> Gain2/1
  Product/1 -> Add/1
  Gain/1 -> Product/2
  Demux/1 -> Product/1
  Product1/1 -> Add/2
  Product2/1 -> Add/3
  Product3/1 -> Add/4
  Demux/2 -> Product1/1
  Demux/3 -> Product2/1
  Demux/4 -> Product3/1
  [Tx] -> Product1/2
  [Ty] -> Product2/2
  Gain2/1 -> Product3/2
  Gain7/1 -> Product7/2
  [Ty] -> Product6/2
  [Tx] -> Product5/2
  Demux1/4 -> Product7/1
  Demux1/3 -> Product6/1
  Demux1/2 -> Product5/1
  Product7/1 -> Add1/4
  Product6/1 -> Add1/3
  Product5/1 -> Add1/2
  Demux1/1 -> Product4/1
  Gain5/1 -> Product4/2
  Product4/1 -> Add1/1
  [Tz] -> Gain7/1
  Add1/1 -> Gain6/1
  [Tz] -> Gain5/1
  [s_seq] -> Demux1/1
  Gain6/1 -> cmp_s/1
  [t_seq] -> Demux2/1
  [Tz] -> Gain10/1
  Add2/1 -> Gain11/1
  [Tz] -> Gain12/1
  Product8/1 -> Add2/1
  Gain10/1 -> Product8/2
  Demux2/1 -> Product8/1
  Product9/1 -> Add2/2
  Product10/1 -> Add2/3
  Product11/1 -> Add2/4
  Demux2/2 -> Product9/1
  Demux2/3 -> Product10/1
  Demux2/4 -> Product11/1
  [Tx] -> Product9/2
  [Ty] -> Product10/2
  Gain12/1 -> Product11/2
  Gain11/1 -> cmp_t/1
  t_seq/1 -> [t_seq]
  s_seq/1 -> [s_seq]

== system npc_controller/CONTROL/SVPWM/SVPWM_with_bal/calcDwellingTimes ==
  Tsw : Inport  OutDataTypeStr=double  PortDimensions=1
  vref_fict_mag_alpha : Inport  Port=2  OutDataTypeStr=double  PortDimensions=1
  vref_fict_mag_beta : Inport  Port=3  OutDataTypeStr=double  PortDimensions=1
  vx_fict_mag_alpha : Inport  Port=4  OutDataTypeStr=double  PortDimensions=1
  vx_fict_mag_beta : Inport  Port=5  OutDataTypeStr=double  PortDimensions=1
  vy_fict_mag_alpha : Inport  Port=6  OutDataTypeStr=double  PortDimensions=1
  vy_fict_mag_beta : Inport  Port=7  OutDataTypeStr=double  PortDimensions=1
  f : TriggerPort  TriggerType=function-call  VariantControl=(inherit)
      settings: CopyFcn=Stateflow.SLINSF.SimulinkMan.removeBlockPreDeleteFcn  PreDeleteFcn=Stateflow.SLINSF.SimulinkMan.unsafePredeleteFcn
  Add : Sum  Inputs=+-
  Add1 : Sum  Inputs=+--
  Cast To Single : DataTypeConversion  OutDataTypeStr=single  SaturateOnIntegerOverflow=off  RndMeth=Floor
  Cast To Single1 : DataTypeConversion  OutDataTypeStr=single  SaturateOnIntegerOverflow=off  RndMeth=Floor
  Cast To Single2 : DataTypeConversion  OutDataTypeStr=single  SaturateOnIntegerOverflow=off  RndMeth=Floor
  Display{,1..17} (18 alike) : Display
  Divide : Product  Inputs=**/
  Divide1 : Product  Inputs=*/
  Product{,1..5} (6 alike) : Product
  Subtract : Sum  Inputs=+-
  Subtract1 : Sum  Inputs=+-
  Tx : Outport
  Ty : Outport  Port=2
  Tz : Outport  Port=3
  wires:
  [vx_fict_mag_beta] -> Product2/1
  [vy_fict_mag_alpha] -> Product2/2
  [Tsw] -> Display17/1, Divide/1
  Cast To Single2/1 -> Tz/1
  Cast To Single1/1 -> Ty/1
  Cast To Single/1 -> Tx/1
  [Tsw] -> Add1/1
  [Tx] -> Add1/2
  [Ty] -> Add1/3
  [vy_fict_mag_alpha] -> Divide1/2
  Subtract1/1 -> Divide1/1
  Product5/1 -> Subtract1/2
  [Tx] -> Product5/2
  [vx_fict_mag_alpha] -> Product5/1
  [Tsw] -> Product4/2
  [vref_fict_mag_alpha] -> Product4/1
  Product4/1 -> Subtract1/1, Display/1
  Subtract/1 -> Display16/1, Divide/3
  Add/1 -> Display11/1, Divide/2
  Product3/1 -> Display14/1, Subtract/2
  Product2/1 -> Display15/1, Subtract/1
  Product1/1 -> Display13/1, Add/2
  Product/1 -> Display12/1, Add/1
  [vy_fict_mag_beta] -> Product3/2
  [vx_fict_mag_alpha] -> Product3/1
  [vy_fict_mag_beta] -> Product1/2
  [vref_fict_mag_alpha] -> Product1/1
  [vy_fict_mag_alpha] -> Product/2
  [vref_fict_mag_beta] -> Product/1
  vy_fict_mag_beta/1 -> [vy_fict_mag_beta], Display10/1
  vy_fict_mag_alpha/1 -> [vy_fict_mag_alpha], Display9/1
  vx_fict_mag_beta/1 -> [vx_fict_mag_beta], Display8/1
  vx_fict_mag_alpha/1 -> [vx_fict_mag_alpha], Display7/1
  vref_fict_mag_beta/1 -> [vref_fict_mag_beta], Display6/1
  vref_fict_mag_alpha/1 -> [vref_fict_mag_alpha], Display5/1
  Tsw/1 -> [Tsw], Display4/1
  Divide/1 -> [Tx], Display1/1, Cast To Single/1
  Divide1/1 -> Cast To Single1/1, [Ty], Display2/1
  Add1/1 -> Cast To Single2/1, Display3/1

== system npc_controller/CONTROL/SVPWM/SVPWM_with_bal/detSeq ==
  subsector : Inport  OutDataTypeStr=double  PortDimensions=1
  f : TriggerPort  TriggerType=function-call  VariantControl=(inherit)
      settings: CopyFcn=Stateflow.SLINSF.SimulinkMan.removeBlockPreDeleteFcn  PreDeleteFcn=Stateflow.SLINSF.SimulinkMan.unsafePredeleteFcn
  Cast To Double : DataTypeConversion  OutDataTypeStr=double  SaturateOnIntegerOverflow=off  RndMeth=Floor
  Cast To Double1 : DataTypeConversion  OutDataTypeStr=double  SaturateOnIntegerOverflow=off  RndMeth=Floor
  Cast To Double2 : DataTypeConversion  OutDataTypeStr=double  SaturateOnIntegerOverflow=off  RndMeth=Floor
  Constant : Constant  Value=[0 1 1 1]
  Constant1 : Constant  Value=[1 1 0 0]
  Constant10 : Constant  Value=[0 0 0 1]
  Constant11 : Constant  Value=[1 0 0 0]
  Constant12 : Constant  Value=[0 1 1 1]
  Constant13 : Constant  Value=[1 1 0 0]
  Constant14 : Constant  Value=[0 0 0 1]
  Constant15 : Constant  Value=[1 0 0 0]
  Constant16 : Constant  Value=[0 0 1 1]
  Constant17 : Constant  Value=[1 1 1 0]
  Constant2 : Constant  Value=[0 0 0 1]
  Constant3 : Constant  Value=[1 0 0 0]
  Constant4 : Constant  Value=[0 0 1 1]
  Constant5 : Constant  Value=[1 1 1 0]
  Constant6 : Constant  Value=[0 0 1 1]
  Constant7 : Constant  Value=[1 1 1 0]
  Constant8 : Constant  Value=[0 1 1 1]
  Constant9 : Constant  Value=[1 1 0 0]
  Multiport Switch : MultiPortSwitch  Inputs=6  DataPortForDefault=Additional data port  SaturateOnIntegerOverflow=off  InputSameDT=off
  Multiport Switch1 : MultiPortSwitch  Inputs=6  DataPortForDefault=Additional data port  SaturateOnIntegerOverflow=off  InputSameDT=off
  Multiport Switch2 : MultiPortSwitch  Inputs=6  DataPortForDefault=Additional data port  SaturateOnIntegerOverflow=off  InputSameDT=off
  r_seq : Outport
  s_seq : Outport  Port=2
  t_seq : Outport  Port=3
  wires:
  Cast To Double2/1 -> t_seq/1
  Cast To Double1/1 -> s_seq/1
  Cast To Double/1 -> r_seq/1
  Multiport Switch/1 -> Cast To Double/1
  subsector/1 -> [subsector]
  [subsector] -> Multiport Switch/1
  Constant/1 -> Multiport Switch/2
  Constant5/1 -> Multiport Switch/7
  Constant4/1 -> Multiport Switch/6
  Constant3/1 -> Multiport Switch/5
  Constant2/1 -> Multiport Switch/4
  Constant1/1 -> Multiport Switch/3
  Constant7/1 -> Multiport Switch1/3
  Constant8/1 -> Multiport Switch1/4
  Constant9/1 -> Multiport Switch1/5
  Constant10/1 -> Multiport Switch1/6
  Constant11/1 -> Multiport Switch1/7
  Constant6/1 -> Multiport Switch1/2
  [subsector] -> Multiport Switch1/1
  Multiport Switch1/1 -> Cast To Double1/1
  [subsector] -> Multiport Switch2/1
  Constant14/1 -> Multiport Switch2/2
  Constant13/1 -> Multiport Switch2/7
  Constant12/1 -> Multiport Switch2/6
  Constant17/1 -> Multiport Switch2/5
  Constant16/1 -> Multiport Switch2/4
  Constant15/1 -> Multiport Switch2/3
  Multiport Switch2/1 -> Cast To Double2/1

== system npc_controller/CONTROL/SVPWM/SVPWM_with_bal/detSeqFixedSmallVector ==
  subsector : Inport  OutDataTypeStr=double  PortDimensions=1
  f : TriggerPort  TriggerType=function-call  VariantControl=(inherit)
      settings: CopyFcn=Stateflow.SLINSF.SimulinkMan.removeBlockPreDeleteFcn  PreDeleteFcn=Stateflow.SLINSF.SimulinkMan.unsafePredeleteFcn
  Cast To Double : DataTypeConversion  OutDataTypeStr=double  SaturateOnIntegerOverflow=off  RndMeth=Floor
  Cast To Double1 : DataTypeConversion  OutDataTypeStr=double  SaturateOnIntegerOverflow=off  RndMeth=Floor
  Cast To Double2 : DataTypeConversion  OutDataTypeStr=double  SaturateOnIntegerOverflow=off  RndMeth=Floor
  Constant{,7..8,12,17} (5 alike) : Constant  Value=[0 1 1 1]
  Constant1 : Constant  Value=[1 1 0 0]
  Constant{2,10..11,14..15} (5 alike) : Constant  Value=[0 0 0 1]
  Constant13 : Constant  Value=[0 1 0 1]
  Constant16 : Constant  Value=[0 0 1 1]
  Constant18 : Constant  Commented=on  Value=[1 1 0 0]
  Constant19 : Constant  Commented=on  Value=[1 0 0 0]
  Constant20 : Constant  Commented=on  Value=[1 1 1 0]
  Constant21 : Constant  Commented=on  Value=[1 1 1 0]
  Constant22 : Constant  Commented=on  Value=[1 1 0 0]
  Constant23 : Constant  Commented=on  Value=[1 0 0 0]
  Constant24 : Constant  Commented=on  Value=[1 0 0 0]
  Constant25 : Constant  Commented=on  Value=[1 1 1 0]
  Constant26 : Constant  Commented=on  Value=[1 1 0 0]
  Constant3 : Constant  Value=[1 0 0 0]
  Constant4 : Constant  Value=[0 0 1 1]
  Constant5 : Constant  Value=[1 1 1 0]
  Constant6 : Constant  Value=[0 0 1 1]
  Constant9 : Constant  Value=[0 1 0 1]
  Multiport Switch : MultiPortSwitch  Inputs=6  DataPortForDefault=Additional data port  SaturateOnIntegerOverflow=off  InputSameDT=off
  Multiport Switch1 : MultiPortSwitch  Inputs=6  DataPortForDefault=Additional data port  SaturateOnIntegerOverflow=off  InputSameDT=off
  Multiport Switch2 : MultiPortSwitch  Inputs=6  DataPortForDefault=Additional data port  SaturateOnIntegerOverflow=off  InputSameDT=off
  r_seq : Outport
  s_seq : Outport  Port=2
  t_seq : Outport  Port=3
  wires:
  Cast To Double2/1 -> t_seq/1
  Cast To Double1/1 -> s_seq/1
  Cast To Double/1 -> r_seq/1
  Multiport Switch/1 -> Cast To Double/1
  subsector/1 -> [subsector]
  [subsector] -> Multiport Switch/1
  Constant/1 -> Multiport Switch/2
  Constant5/1 -> Multiport Switch/7
  Constant4/1 -> Multiport Switch/6
  Constant3/1 -> Multiport Switch/5
  Constant2/1 -> Multiport Switch/4
  Constant1/1 -> Multiport Switch/3
  Constant7/1 -> Multiport Switch1/3
  Constant8/1 -> Multiport Switch1/4
  Constant9/1 -> Multiport Switch1/5
  Constant10/1 -> Multiport Switch1/6
  Constant11/1 -> Multiport Switch1/7
  Constant6/1 -> Multiport Switch1/2
  [subsector] -> Multiport Switch1/1
  Multiport Switch1/1 -> Cast To Double1/1
  [subsector] -> Multiport Switch2/1
  Constant14/1 -> Multiport Switch2/2
  Constant13/1 -> Multiport Switch2/7
  Constant12/1 -> Multiport Switch2/6
  Constant17/1 -> Multiport Switch2/5
  Constant16/1 -> Multiport Switch2/4
  Constant15/1 -> Multiport Switch2/3
  Multiport Switch2/1 -> Cast To Double2/1

== system npc_controller/CONTROL/SVPWM/Subsystem ==
  Trigger : TriggerPort  TriggerType=function-call  VariantControl=Variant  PortDimensions=1
  Constant16 : Constant
  Out1 : Outport
  wires:
  Constant16/1 -> Out1/1

== system npc_controller/CONTROL/SVPWM/Subsystem1 ==
  note: interacting PID
  error : Inport
  disable : Inport  Port=2
  Constant : Constant  Value=18.57
  Constant1 : Constant  Value=-34.95
  Constant2 : Constant  Value=470
  Constant3 : Constant  Value=-470
  Constant4 : Constant  Value=16.46
  Constant5 : Constant  Value=-1.246
  Constant6 : Constant  Value=0.2457
  Delay{1..4} (4 alike) : Delay  DelayLength=1  InitialCondition=0  ExternalReset=Level
      settings: InputPortMap=u0,r5
  Product{1..5} (5 alike) : Product
  Saturation Dynamic1 : simulink/Discontinuities/Saturation Dynamic  OutMin=[]  OutMax=[]  OutDataTypeStr=double  OutputDataTypeScalingMode=double  OutDataType=fixdt(1, 16)  OutScaling=2^-10  DoSatur=off
  Scope : Scope  NumInputPorts=4
  Sum : Sum  Inputs=|+++--
  pi : Outport
  wires:
  [error] -> Scope/1  "error"
  [kP_term] -> Scope/2  "kP_term"
  [kI_term] -> Scope/3  "kI_term"
  [pi] -> Scope/4  "PI"
  [a0] -> Product3/2
  Sum/1 -> Saturation Dynamic1/2
  [integ_min] -> Saturation Dynamic1/3
  [integ_max] -> Saturation Dynamic1/1
  Constant2/1 -> [integ_max]
  Constant3/1 -> [integ_min]
  Constant1/1 -> [a1]
  error/1 -> [error]
  [a1] -> Product2/2
  Constant/1 -> [a0]
  [error] -> Delay2/1, Product3/1
  Delay2/1 -> Product2/1, Delay3/1
  Saturation Dynamic1/1 -> pi/1, Delay1/1, [pi]
  Delay3/1 -> Product1/1
  [a2] -> Product1/2
  Product3/1 -> Sum/1
  Product2/1 -> Sum/2
  Product1/1 -> Sum/3
  Delay1/1 -> Product4/2, Delay4/1
  [b1] -> Product4/1
  Delay4/1 -> Product5/2
  Product5/1 -> Sum/5
  Product4/1 -> Sum/4
  [b2] -> Product5/1
  Constant5/1 -> [b1]
  Constant4/1 -> [a2]
  Constant6/1 -> [b2]
  disable/1 -> Delay4/2, Delay1/2, Delay3/2, Delay2/2

== system npc_controller/CONTROL/SVPWM/Subsystem2 ==
  note: Parallel PI
  error : Inport
  Constant : Constant  Value=0.3055
  Constant1 : Constant  Value=-0.3052
  Constant2 : Constant  Value=50
  Constant3 : Constant  Value=-50
  Constant4 : Constant  Commented=on  Value=36
  Constant5 : Constant  Commented=on  Value=-36
  Constant6 : Constant  Commented=on  Value=0.611
  Constant7 : Constant  Commented=on  Value=-0.6105
  Delay1 : Delay  DelayLength=1  InitialCondition=22
  Delay2 : Delay  DelayLength=1  InitialCondition=0
  Product2 : Product
  Product3 : Product
  Saturation Dynamic1 : simulink/Discontinuities/Saturation Dynamic  OutMin=[]  OutMax=[]  OutDataTypeStr=double  OutputDataTypeScalingMode=double  OutDataType=fixdt(1, 16)  OutScaling=2^-10  DoSatur=off
  Scope : Scope  NumInputPorts=4
  Sum : Sum  Inputs=|++
  Sum3 : Sum  Inputs=|++
  pi : Outport
  wires:
  Saturation Dynamic1/1 -> [pi], Delay1/1, pi/1
  Delay2/1 -> Product2/1
  [error] -> Delay2/1
  Sum3/1 -> Sum/2, [kI_term]
  Delay1/1 -> Sum3/2
  Constant/1 -> [kp]
  [ki] -> Product2/2
  error/1 -> [error]
  Constant1/1 -> [ki]
  [error] -> Product3/1
  Product3/1 -> [kP_term], Sum/1
  Product2/1 -> Sum3/1
  Constant3/1 -> [integ_min]
  Constant2/1 -> [integ_max]
  [integ_max] -> Saturation Dynamic1/1
  [integ_min] -> Saturation Dynamic1/3
  Sum/1 -> Saturation Dynamic1/2
  [kp] -> Product3/2
  [pi] -> Scope/4  "PI"
  [kI_term] -> Scope/3  "kI_term"
  [kP_term] -> Scope/2  "kP_term"
  [error] -> Scope/1  "error"

== system npc_controller/CONTROL/SVPWM/Subsystem4 ==
  note: interacting PID
  error : Inport
  disable : Inport  Port=2
  Constant : Constant  Value=18.57
  Constant1 : Constant  Value=-34.95
  Constant2 : Constant  Value=470
  Constant3 : Constant  Value=-470
  Constant4 : Constant  Value=16.46
  Constant5 : Constant  Value=-1.246
  Constant6 : Constant  Value=0.2457
  Delay{1..4} (4 alike) : Delay  DelayLength=1  InitialCondition=0  ExternalReset=Level
      settings: InputPortMap=u0,r5
  Product{1..5} (5 alike) : Product
  Saturation Dynamic1 : simulink/Discontinuities/Saturation Dynamic  OutMin=[]  OutMax=[]  OutDataTypeStr=double  OutputDataTypeScalingMode=double  OutDataType=fixdt(1, 16)  OutScaling=2^-10  DoSatur=off
  Scope : Scope  NumInputPorts=4
  Sum : Sum  Inputs=|+++--
  pi : Outport
  wires:
  disable/1 -> Delay2/2, Delay3/2, Delay1/2, Delay4/2
  Constant6/1 -> [b2]
  Constant4/1 -> [a2]
  Constant5/1 -> [b1]
  [b2] -> Product5/1
  Product4/1 -> Sum/4
  Product5/1 -> Sum/5
  Delay4/1 -> Product5/2
  [b1] -> Product4/1
  Delay1/1 -> Delay4/1, Product4/2
  Product1/1 -> Sum/3
  Product2/1 -> Sum/2
  Product3/1 -> Sum/1
  [a2] -> Product1/2
  Delay3/1 -> Product1/1
  Saturation Dynamic1/1 -> [pi], Delay1/1, pi/1
  Delay2/1 -> Delay3/1, Product2/1
  [error] -> Product3/1, Delay2/1
  Constant/1 -> [a0]
  [a1] -> Product2/2
  error/1 -> [error]
  Constant1/1 -> [a1]
  Constant3/1 -> [integ_min]
  Constant2/1 -> [integ_max]
  [integ_max] -> Saturation Dynamic1/1
  [integ_min] -> Saturation Dynamic1/3
  Sum/1 -> Saturation Dynamic1/2
  [a0] -> Product3/2
  [pi] -> Scope/4  "PI"
  [kI_term] -> Scope/3  "kI_term"
  [kP_term] -> Scope/2  "kP_term"
  [error] -> Scope/1  "error"

== system npc_controller/CONTROL/SVPWM/Subsystem5 ==
  note: Parallel PI
  error : Inport
  Constant : Constant  Value=0.611e-1
  Constant1 : Constant  Value=-0.6105e-1
  Constant2 : Constant  Value=0.8
  Constant3 : Constant  Value=0.2
  Constant4 : Constant  Commented=on  Value=36
  Constant5 : Constant  Commented=on  Value=-36
  Constant6 : Constant  Commented=on  Value=0.611e-1
  Constant7 : Constant  Commented=on  Value=-0.6105e-1
  Delay1 : Delay  DelayLength=1  InitialCondition=22
  Delay2 : Delay  DelayLength=1  InitialCondition=0
  Product2 : Product
  Product3 : Product
  Saturation Dynamic1 : simulink/Discontinuities/Saturation Dynamic  OutMin=[]  OutMax=[]  OutDataTypeStr=double  OutputDataTypeScalingMode=double  OutDataType=fixdt(1, 16)  OutScaling=2^-10  DoSatur=off
  Scope : Scope  NumInputPorts=4
  Sum : Sum  Inputs=|++
  Sum3 : Sum  Inputs=|++
  pi : Outport
  wires:
  Saturation Dynamic1/1 -> [pi], Delay1/1, pi/1
  Delay2/1 -> Product2/1
  [error] -> Delay2/1
  Sum3/1 -> Sum/2, [kI_term]
  Delay1/1 -> Sum3/2
  Constant/1 -> [kp]
  [ki] -> Product2/2
  error/1 -> [error]
  Constant1/1 -> [ki]
  [error] -> Product3/1
  Product3/1 -> [kP_term], Sum/1
  Product2/1 -> Sum3/1
  Constant3/1 -> [integ_min]
  Constant2/1 -> [integ_max]
  [integ_max] -> Saturation Dynamic1/1
  [integ_min] -> Saturation Dynamic1/3
  Sum/1 -> Saturation Dynamic1/2
  [kp] -> Product3/2
  [pi] -> Scope/4  "PI"
  [kI_term] -> Scope/3  "kI_term"
  [kP_term] -> Scope/2  "kP_term"
  [error] -> Scope/1  "error"

== system npc_controller/CONTROL/SVPWM/Subsystem6 ==
  note: Parallel PI
  error : Inport
  Constant : Constant  Value=1.407
  Constant1 : Constant  Value=-1.387
  Constant2 : Constant  Value=470
  Constant3 : Constant  Value=-470
  Constant4 : Constant  Commented=on  Value=470
  Constant5 : Constant  Commented=on  Value=-470
  Constant6 : Constant  Commented=on  Value=0.7034
  Constant7 : Constant  Commented=on  Value=-0.6871
  Delay1 : Delay  DelayLength=1  InitialCondition=0
  Delay2 : Delay  DelayLength=1  InitialCondition=0
  Product2 : Product
  Product3 : Product
  Saturation Dynamic1 : simulink/Discontinuities/Saturation Dynamic  OutMin=[]  OutMax=[]  OutDataTypeStr=double  OutputDataTypeScalingMode=double  OutDataType=fixdt(1, 16)  OutScaling=2^-10  DoSatur=off
  Scope : Scope  NumInputPorts=4
  Sum : Sum  Inputs=|++
  Sum3 : Sum  Inputs=|++
  pi : Outport
  wires:
  [error] -> Scope/1  "error"
  [kP_term] -> Scope/2  "kP_term"
  [kI_term] -> Scope/3  "kI_term"
  [pi] -> Scope/4  "PI"
  [kp] -> Product3/2
  Sum/1 -> Saturation Dynamic1/2
  [integ_min] -> Saturation Dynamic1/3
  [integ_max] -> Saturation Dynamic1/1
  Constant2/1 -> [integ_max]
  Constant3/1 -> [integ_min]
  Product2/1 -> Sum3/1
  Product3/1 -> Sum/1, [kP_term]
  [error] -> Product3/1
  Constant1/1 -> [ki]
  error/1 -> [error]
  [ki] -> Product2/2
  Constant/1 -> [kp]
  Delay1/1 -> Sum3/2
  Sum3/1 -> [kI_term], Sum/2
  [error] -> Delay2/1
  Delay2/1 -> Product2/1
  Saturation Dynamic1/1 -> pi/1, Delay1/1, [pi]

== system npc_controller/CONTROL/SVPWM/Subsystem7 ==
  note: Parallel PI
  error : Inport
  Constant : Constant  Value=1.407
  Constant1 : Constant  Value=-1.387
  Constant2 : Constant  Value=470
  Constant3 : Constant  Value=-470
  Constant4 : Constant  Commented=on  Value=470
  Constant5 : Constant  Commented=on  Value=-470
  Constant6 : Constant  Commented=on  Value=0.7034
  Constant7 : Constant  Commented=on  Value=-0.6871
  Delay1 : Delay  DelayLength=1  InitialCondition=0
  Delay2 : Delay  DelayLength=1  InitialCondition=0
  Product2 : Product
  Product3 : Product
  Saturation Dynamic1 : simulink/Discontinuities/Saturation Dynamic  OutMin=[]  OutMax=[]  OutDataTypeStr=double  OutputDataTypeScalingMode=double  OutDataType=fixdt(1, 16)  OutScaling=2^-10  DoSatur=off
  Scope : Scope  NumInputPorts=4
  Sum : Sum  Inputs=|++
  Sum3 : Sum  Inputs=|++
  pi : Outport
  wires:
  [error] -> Scope/1  "error"
  [kP_term] -> Scope/2  "kP_term"
  [kI_term] -> Scope/3  "kI_term"
  [pi] -> Scope/4  "PI"
  [kp] -> Product3/2
  Sum/1 -> Saturation Dynamic1/2
  [integ_min] -> Saturation Dynamic1/3
  [integ_max] -> Saturation Dynamic1/1
  Constant2/1 -> [integ_max]
  Constant3/1 -> [integ_min]
  Product2/1 -> Sum3/1
  Product3/1 -> Sum/1, [kP_term]
  [error] -> Product3/1
  Constant1/1 -> [ki]
  error/1 -> [error]
  [ki] -> Product2/2
  Constant/1 -> [kp]
  Delay1/1 -> Sum3/2
  Sum3/1 -> [kI_term], Sum/2
  [error] -> Delay2/1
  Delay2/1 -> Product2/1
  Saturation Dynamic1/1 -> pi/1, Delay1/1, [pi]

== system npc_controller/CONTROL/SVPWM/abc to dq ==
  note: wt
  note: wt
  note: wt
  note: wt
  note: wt
  note: wt
  abc : Inport
  wt : Inport  Port=2
  (wt+120) : Sum  Inputs=|++
  (wt-120) : Sum  Inputs=|+-
  2pi_3 : Constant  Value=2*pi/3
  Add2 : Sum  Inputs=+++
  Add3 : Sum  Inputs=+++
  Cos : Trigonometry
  Cos1 : Trigonometry
  Cos2 : Trigonometry
  Cos3 : Trigonometry  Operator=cos
  Cos4 : Trigonometry  Operator=cos
  Cos5 : Trigonometry  Operator=cos
  Demux : Demux  Outputs=3
  Mux : Mux  Inputs=3
  Product{2..7} (6 alike) : Product
  d1 : Gain  Gain=2/3
  q1 : Gain  Gain=2/3
  wt+120 : Sum  Inputs=|++
  wt-120 : Sum  Inputs=|+-
  dq0 : Outport
  wires:
  Mux/1 -> dq0/1
  abc/1 -> Demux/1
  2pi_3/1 -> [ph]
  q1/1 -> Mux/2
  [c] -> Product7/1
  Add3/1 -> q1/1
  [c] -> Product4/1
  wt-120/1 -> Cos1/1
  Demux/2 -> [b]
  [ph] -> wt-120/2
  Cos2/1 -> Product4/2
  wt+120/1 -> Cos2/1
  Cos5/1 -> Product7/2
  [ph] -> wt+120/2
  d1/1 -> Mux/1
  [b] -> Product3/1
  Product5/1 -> Add3/1
  Cos4/1 -> Product6/2
  [b] -> Product6/1
  (wt-120)/1 -> Cos4/1
  [ph] -> (wt-120)/2
  Demux/3 -> [c]
  Product6/1 -> Add3/2
  Product2/1 -> Add2/1
  (wt+120)/1 -> Cos5/1
  Product4/1 -> Add2/3
  Demux/1 -> [a]
  Product7/1 -> Add3/3
  [ph] -> (wt+120)/2
  Add2/1 -> d1/1
  wt/1 -> Cos3/1, (wt-120)/1, (wt+120)/1, wt+120/1, Cos/1, wt-120/1
  Product3/1 -> Add2/2
  [a] -> Product2/1
  Cos1/1 -> Product3/2
  Cos3/1 -> Product5/2
  Cos/1 -> Product2/2
  [a] -> Product5/1

== system npc_controller/CONTROL/SVPWM/abc to dq1 ==
  note: wt
  note: wt
  note: wt
  note: wt
  note: wt
  note: wt
  abc : Inport
  wt : Inport  Port=2
  (wt+120) : Sum  Inputs=|++
  (wt-120) : Sum  Inputs=|+-
  2pi_3 : Constant  Value=2*pi/3
  Add2 : Sum  Inputs=+++
  Add3 : Sum  Inputs=+++
  Cos : Trigonometry
  Cos1 : Trigonometry
  Cos2 : Trigonometry
  Cos3 : Trigonometry  Operator=cos
  Cos4 : Trigonometry  Operator=cos
  Cos5 : Trigonometry  Operator=cos
  Demux : Demux  Outputs=3
  Mux : Mux  Inputs=3
  Product{2..7} (6 alike) : Product
  d1 : Gain  Gain=2/3
  q1 : Gain  Gain=2/3
  wt+120 : Sum  Inputs=|++
  wt-120 : Sum  Inputs=|+-
  dq0 : Outport
  wires:
  [a] -> Product5/1
  Cos/1 -> Product2/2
  Cos3/1 -> Product5/2
  Cos1/1 -> Product3/2
  [a] -> Product2/1
  Product3/1 -> Add2/2
  wt/1 -> wt-120/1, Cos/1, wt+120/1, (wt+120)/1, (wt-120)/1, Cos3/1
  Add2/1 -> d1/1
  [ph] -> (wt+120)/2
  Product7/1 -> Add3/3
  Demux/1 -> [a]
  Product4/1 -> Add2/3
  (wt+120)/1 -> Cos5/1
  Product2/1 -> Add2/1
  Product6/1 -> Add3/2
  Demux/3 -> [c]
  [ph] -> (wt-120)/2
  (wt-120)/1 -> Cos4/1
  [b] -> Product6/1
  Cos4/1 -> Product6/2
  Product5/1 -> Add3/1
  [b] -> Product3/1
  d1/1 -> Mux/1
  [ph] -> wt+120/2
  Cos5/1 -> Product7/2
  wt+120/1 -> Cos2/1
  Cos2/1 -> Product4/2
  [ph] -> wt-120/2
  Demux/2 -> [b]
  wt-120/1 -> Cos1/1
  [c] -> Product4/1
  Add3/1 -> q1/1
  [c] -> Product7/1
  q1/1 -> Mux/2
  2pi_3/1 -> [ph]
  abc/1 -> Demux/1
  Mux/1 -> dq0/1
